simulink library "DABLib"  (R2016b)
settings: Solver=VariableStepAuto  StartTime=0.0  StopTime=10.0  RelTol=1e-3
undefined symbols (not defined in the file or in its folder): ln, sgn
libraries: DABLib x53, simulink_extras x2, simulink x1
(part 3 of 3)

== system DABLib/DABLibUtil/CoreAct/Ps//X transducer Pneumatic servo-motor/Twisted servomotor's rod fault f8 ==
  note: Fault  f8
      | Twisted servomotor's fault
      | simulated as linear function of X
  Db[m] : Inport
  X[%] : Inport  Port=2
  f8<0,1> : Inport  Port=3
  " " : Fcn  Expr=u(1)*(1+u(2)*u(3)*(1-u(4)))
  "Deadband 0..0.0381m " : Saturate  UpperLimit=0.0381  LowerLimit=0
  "Fault streght saturation 0..100% " : Saturate  UpperLimit=1.0  LowerLimit=0
  Higher bound 0..0.0381 : Saturate  UpperLimit=0.0381  LowerLimit=0
  Hysteresis change range in [%] : Constant  Value=0.5
  Mux4 : Mux
  Dbf[m] : Outport
  wires:
  " "/1 -> "Deadband 0..0.0381m "/1
  X[%]/1 -> Mux4/4
  Mux4/1 -> " "/1
  "Deadband 0..0.0381m "/1 -> Dbf[m]/1
  "Fault streght saturation 0..100% "/1 -> Mux4/3
  f8<0,1>/1 -> "Fault streght saturation 0..100% "/1
  Higher bound 0..0.0381/1 -> Mux4/1
  Db[m]/1 -> Higher bound 0..0.0381/1
  Hysteresis change range in [%]/1 -> Mux4/2

== system DABLib/DABLibUtil/CoreAct/Ps//X transducer Pneumatic servo-motor/Valve clogging fault f1 ==
  note: Fault  f1
      | Valve clogging fault
  Hb[m] : Inport
  f1<0,1> : Inport  Port=2
  " " : Fcn  Expr=u(1)*(1-u(2))
  "Fault streght saturation 0..100% " : Saturate  UpperLimit=1.0  LowerLimit=0
  Higher bound limit 0..0.0381m : Saturate  UpperLimit=0.0381  LowerLimit=0
  "Higher bound limit 0..0.0381m " : Saturate  UpperLimit=0.0381  LowerLimit=0
  Mux4 : Mux  Inputs=2
  Hbf[m] : Outport
  wires:
  "Fault streght saturation 0..100% "/1 -> Mux4/2
  Higher bound limit 0..0.0381m/1 -> Mux4/1
  Hb[m]/1 -> Higher bound limit 0..0.0381m/1
  " "/1 -> "Higher bound limit 0..0.0381m "/1
  Mux4/1 -> " "/1
  "Higher bound limit 0..0.0381m "/1 -> Hbf[m]/1
  f1<0,1>/1 -> "Fault streght saturation 0..100% "/1

== system DABLib/DABLibUtil/CoreAct/Ps//X transducer Pneumatic servo-motor/Valve errossion fault f3 ==
  note: Fault  f3
      | Valve plug or valve seat
      | errosion fault
  Hb[m] : Inport
  f3<0,1> : Inport  Port=2
  " " : Fcn  Expr=u(1)*(1+u(2)*u(3))
  Errossion relative span : Constant  Value=0.1
  "Fault streght saturation 0..100% " : Saturate  UpperLimit=1.0  LowerLimit=-1.0
  Higher bound limit 0..0.0381m : Saturate  UpperLimit=0.0381  LowerLimit=0
  "Higher bound limit 0..inf " : Saturate  UpperLimit=inf  LowerLimit=0
  Mux4 : Mux  Inputs=3
  Hbf[m] : Outport
  wires:
  Errossion relative span/1 -> Mux4/2
  "Fault streght saturation 0..100% "/1 -> Mux4/3
  Higher bound limit 0..0.0381m/1 -> Mux4/1
  Hb[m]/1 -> Higher bound limit 0..0.0381m/1
  " "/1 -> "Higher bound limit 0..inf "/1
  Mux4/1 -> " "/1
  "Higher bound limit 0..inf "/1 -> Hbf[m]/1
  f3<0,1>/1 -> "Fault streght saturation 0..100% "/1

== system DABLib/DABLibUtil/CoreAct/Ps//X transducer Pneumatic servo-motor/WUT Backlash ==
  dead band : Inport
  signal : Inport  Port=2
  Hysteresis : Subsystem
  Memory1 : Memory
  WUT direction decoder : Subsystem
  output : Outport
  wires:
  Hysteresis/1(hysta) -> Memory1/1, output/1
  Memory1/1 -> Hysteresis/4(history)
  dead band/1 -> Hysteresis/3(h_band)
  WUT direction decoder/1(direction) -> Hysteresis/2(x_dir)
  signal/1 -> Hysteresis/1(x), WUT direction decoder/1("signal ")

== system DABLib/DABLibUtil/CoreAct/Water flow control valve/Equipercentage rated flow coefficient ==
  note: Equipercentage rated flow
      | coefficient
  X[%] : Inport
  " 1" : Sum  Inputs=+-  SaturateOnIntegerOverflow=on  InputSameDT=on  OutDataTypeStr=Inherit: Same as first input
  " Valve Kv exponent" : Constant  Value=5
  Comparator : RelationalOperator  Operator=>  RndMeth=Nearest  InputSameDT=on
  End of equipercentage characteristics : Constant  Value=0.975
  Mux8 : Mux  Inputs=2
  Mux9 : Mux
  Rated flow coefficient Kv[%]=f(X[%]) Equipercentage part : Fcn  Expr=exp(u(2)*(1-u(1)))/exp(u(2))
  Rated flow coefficient Kv[%]=f[X[%]) Linear part : Fcn  Expr=u(2)*(u(4)-u(3))*(u(1)/(1-u(3)))
  Saturation 0..100% : Saturate  UpperLimit=1.00  LowerLimit=0
  Saturation 0..97.5% : Saturate  UpperLimit=0.975  LowerLimit=0
  Saturation 97.5%..100% : Saturate  UpperLimit=1.000  LowerLimit=0.975
  Kvr[%] : Outport
  wires:
  Saturation 0..100%/1 -> Saturation 97.5%..100%/1, Saturation 0..97.5%/1
  X[%]/1 -> Saturation 0..100%/1
  " 1"/1 -> Kvr[%]/1
  Rated flow coefficient Kv[%]=f[X[%]) Linear part/1 -> " 1"/2
  Saturation 97.5%..100%/1 -> Mux9/4, Comparator/1
  End of equipercentage characteristics/1 -> Mux9/3, Comparator/2
  Rated flow coefficient Kv[%]=f(X[%]) Equipercentage part/1 -> " 1"/1, Mux9/1
  Comparator/1 -> Mux9/2
  Mux9/1 -> Rated flow coefficient Kv[%]=f[X[%]) Linear part/1
  Saturation 0..97.5%/1 -> Mux8/1
  " Valve Kv exponent"/1 -> Mux8/2
  Mux8/1 -> Rated flow coefficient Kv[%]=f(X[%]) Equipercentage part/1

== system DABLib/DABLibUtil/CoreAct/Water flow control valve/Errosion fault  f3 gaining Kvr  ==
  note: Fault  f3
      | Errossion fault
  Kvr[%] : Inport
  f3<0,1> : Inport  Port=2
  " " : Fcn  Expr=u(1)*(1+u(2)*u(3))
  "Fault streght saturation 0..100% " : Saturate  UpperLimit=1.0  LowerLimit=0.0
  Mux4 : Mux  Inputs=3
  "Relative Kvr saturation 0..100% " : Saturate  UpperLimit=1.0  LowerLimit=0.0
  "Seat errosion relative span " : Constant  Value=0.10
  Kvrf[%] : Outport
  wires:
  "Relative Kvr saturation 0..100% "/1 -> Kvrf[%]/1
  " "/1 -> "Relative Kvr saturation 0..100% "/1
  "Seat errosion relative span "/1 -> Mux4/2
  "Fault streght saturation 0..100% "/1 -> Mux4/3
  f3<0,1>/1 -> "Fault streght saturation 0..100% "/1
  Kvr[%]/1 -> Mux4/1
  Mux4/1 -> " "/1

== system DABLib/DABLibUtil/CoreAct/Water flow control valve/Errossion fault  f3 X negative offset ==
  note: Fault  f3
      | Errossion fault
  X[%] : Inport
  f3<0,1> : Inport  Port=2
  " " : Fcn  Expr=u(1)-u(2)*u(3)
  "Fault range " : Constant  Value=0.10
  "Fault streght saturation 0..100% " : Saturate  UpperLimit=1.0  LowerLimit=0.0
  Mux4 : Mux  Inputs=3
  "Relative Xf saturation 0..100% " : Saturate  UpperLimit=1.0  LowerLimit=0.0
  Xf[%] : Outport
  wires:
  "Relative Xf saturation 0..100% "/1 -> Xf[%]/1
  " "/1 -> "Relative Xf saturation 0..100% "/1
  "Fault range "/1 -> Mux4/2
  "Fault streght saturation 0..100% "/1 -> Mux4/3
  f3<0,1>/1 -> "Fault streght saturation 0..100% "/1
  X[%]/1 -> Mux4/1
  Mux4/1 -> " "/1

== system DABLib/DABLibUtil/CoreAct/Water flow control valve/Internal leakage fault  f6 additive fault ==
  note: Fault  f6
      | Internal leakage fault
      | virtual Kv change
  Kvr[%] : Inport
  f6<0,1> : Inport  Port=2
  " " : Fcn  Expr=u(1)+u(2)*u(3)
  Fault range in [%] <0..1> : Constant  Value=0.10
  "Fault streght saturation 0..100% " : Saturate  UpperLimit=1.0  LowerLimit=0.0
  Mux4 : Mux  Inputs=3
  Kvrf[%] : Outport
  wires:
  Fault range in [%] <0..1>/1 -> Mux4/2
  "Fault streght saturation 0..100% "/1 -> Mux4/3
  " "/1 -> Kvrf[%]/1
  f6<0,1>/1 -> "Fault streght saturation 0..100% "/1
  Kvr[%]/1 -> Mux4/1
  Mux4/1 -> " "/1

== system DABLib/DABLibUtil/CoreAct/Water flow control valve/Sedimentation fault  f2 Kvr lowering ==
  note: Fault  f2
      | Sedimentation fault
  Kvr[%] : Inport
  f2<0,1> : Inport  Port=2
  " " : Fcn  Expr=u(1)*(1-u(2)*u(3))
  "Fault streght saturation 0..100% " : Saturate  UpperLimit=1.0  LowerLimit=0.0
  Mux4 : Mux  Inputs=3
  "Relative Kvr saturation 0..100% " : Saturate  UpperLimit=1.0  LowerLimit=0.0
  "Seat sedimentation relative span " : Constant  Value=0.20
  Kvrf[%] : Outport
  wires:
  "Relative Kvr saturation 0..100% "/1 -> Kvrf[%]/1
  " "/1 -> "Relative Kvr saturation 0..100% "/1
  "Seat sedimentation relative span "/1 -> Mux4/2
  "Fault streght saturation 0..100% "/1 -> Mux4/3
  f2<0,1>/1 -> "Fault streght saturation 0..100% "/1
  Kvr[%]/1 -> Mux4/1
  Mux4/1 -> " "/1

== system DABLib/DABLibUtil/CoreAct/Water flow control valve/Sedimentation fault  f2 X positive offset ==
  note: Fault  f2
      | Sedimentation fault
  X[%] : Inport
  f2<0,1> : Inport  Port=2
  " " : Fcn  Expr=u(1)+u(2)*u(3)
  "Fault range " : Constant  Value=0.20
  "Fault streght saturation 0..100% " : Saturate  UpperLimit=1.0  LowerLimit=0.0
  Mux4 : Mux  Inputs=3
  "Relative Xf saturation 0..100% " : Saturate  UpperLimit=1.0  LowerLimit=0.0
  Xf[%] : Outport
  wires:
  "Relative Xf saturation 0..100% "/1 -> Xf[%]/1
  " "/1 -> "Relative Xf saturation 0..100% "/1
  "Fault range "/1 -> Mux4/2
  "Fault streght saturation 0..100% "/1 -> Mux4/3
  f2<0,1>/1 -> "Fault streght saturation 0..100% "/1
  X[%]/1 -> Mux4/1
  Mux4/1 -> " "/1

== system DABLib/DABLibUtil/CoreAct/Water flow control valve/water specific gravity ==
  note: Water specific gravity versus temperature and pressure
  P[Pa] : Inport
  T[C] : Inport  Port=2
  1-C*P : Fcn  Expr=1-u
  C*P : Product  SaturateOnIntegerOverflow=on  RndMeth=Zero  InputSameDT=on  OutDataTypeStr=Inherit: Same as first input
  Switch : Switch  Threshold=30  SaturateOnIntegerOverflow=on  InputSameDT=on
  Temperature range 0..110C : Saturate  UpperLimit=110  LowerLimit=0
  Water compessibility coefficient : Lookup  InputValues=[0 10 20 50 110]  Table="[5.26e-10 5.02e-10  4.81e-10 4.69e-10 4.42e-10]"  SaturateOnIntegerOverflow=on
  "ro(T)/(1-C(T)*P) " : Product  Inputs=*/  SaturateOnIntegerOverflow=on  RndMeth=Zero  InputSameDT=on  OutDataTypeStr=Inherit: Same as first input
  ro[kg/m^3] t<0..40>C : Fcn  Expr=1000-(((u-4)^2)/503570)*(u+283)*1000/(u+67.2)
  ro[kg/m^3] t<25..100>C : Fcn  Expr=1000-((((u-4)^2)/466700)*(u+273)*1000*(350-u))/((u+67)*(365-u))
  ro[kg/m^3] : Outport
  wires:
  "ro(T)/(1-C(T)*P) "/1 -> ro[kg/m^3]/1
  1-C*P/1 -> "ro(T)/(1-C(T)*P) "/2
  Switch/1 -> "ro(T)/(1-C(T)*P) "/1
  C*P/1 -> 1-C*P/1
  Water compessibility coefficient/1 -> C*P/1
  ro[kg/m^3] t<25..100>C/1 -> Switch/1
  ro[kg/m^3] t<0..40>C/1 -> Switch/3
  Temperature range 0..110C/1 -> Water compessibility coefficient/1, Switch/2, ro[kg/m^3] t<0..40>C/1, ro[kg/m^3] t<25..100>C/1
  T[C]/1 -> Temperature range 0..110C/1
  P[Pa]/1 -> C*P/2

== system DABLib/PICalc/Zones Selection/Stop-watch 1st/Stop-watch ==
  Trigger : TriggerPort  VariantControl=Variant  ShowOutputPort=on
  Digital Clock : DigitalClock  SampleTime=-1
  t(k) : Outport  InitialOutput=-1
  TR : Outport  Port=2  InitialOutput=0
  wires:
  Digital Clock/1 -> t(k)/1
  Trigger/1 -> TR/1

== system DABLib/DABLibUtil/CoreAct/Positioner feedback/WUT Backlash/Hysteresis ==
  x : Inport
  x_dir : Inport  Port=2
  h_band : Inport  Port=3
  history : Inport  Port=4
  Gain : Gain  Gain=0.5  SaturateOnIntegerOverflow=on  OutDataTypeStr=Inherit: Same as input  ParamDataTypeStr=Inherit: Same as input
  MinMax : MinMax  Inputs=2  SaturateOnIntegerOverflow=on  InputSameDT=on
  MinMax1 : MinMax  Function=max  Inputs=2  SaturateOnIntegerOverflow=on  InputSameDT=on
  Switch : Switch  Threshold=0.5  SaturateOnIntegerOverflow=on  InputSameDT=on
  sum : Sum  Inputs=+-  SaturateOnIntegerOverflow=on  InputSameDT=on  OutDataTypeStr=Inherit: Same as first input
  sum1 : Sum  SaturateOnIntegerOverflow=on  InputSameDT=on  OutDataTypeStr=Inherit: Same as first input
  hysta : Outport  InitialOutput=0
  wires:
  Gain/1 -> sum/2, sum1/2
  sum1/1 -> MinMax/1  "y"
  history/1 -> MinMax/2, MinMax1/2
  h_band/1 -> Gain/1
  Switch/1 -> hysta/1
  sum/1 -> MinMax1/1  "z"
  x_dir/1 -> Switch/2
  MinMax1/1 -> Switch/1
  MinMax/1 -> Switch/3
  x/1 -> sum/1, sum1/1

== system DABLib/DABLibUtil/CoreAct/Positioner feedback/WUT Backlash/WUT direction decoder ==
  note: du/dt
  "signal " : Inport
  Memory : Memory
  Sum2 : Sum  Inputs=+-  SaturateOnIntegerOverflow=on  InputSameDT=on  OutDataTypeStr=Inherit: Same as first input
  Terminator : Terminator
  Zero cross : HitCross  HitCrossingDirection=falling
  "Zero cross " : HitCross  HitCrossingDirection=rising
  direction FF : simulink_extras/Flip Flops/S-R Flip-Flop  initial_condition=0
  direction : Outport
  wires:
  direction FF/2 -> Terminator/1
  "signal "/1 -> Memory/1, Sum2/1
  direction FF/1 -> direction/1  "u2"
  Sum2/1 -> "Zero cross "/1, Zero cross/1
  Memory/1 -> Sum2/2
  Zero cross/1 -> direction FF/2
  "Zero cross "/1 -> direction FF/1

== system DABLib/DABLibUtil/CoreAct/Ps//X transducer Pneumatic servo-motor/WUT Backlash/Hysteresis ==
  x : Inport
  x_dir : Inport  Port=2
  h_band : Inport  Port=3
  history : Inport  Port=4
  Gain : Gain  Gain=0.5  SaturateOnIntegerOverflow=on  OutDataTypeStr=Inherit: Same as input  ParamDataTypeStr=Inherit: Same as input
  MinMax : MinMax  Inputs=2  SaturateOnIntegerOverflow=on  InputSameDT=on
  MinMax1 : MinMax  Function=max  Inputs=2  SaturateOnIntegerOverflow=on  InputSameDT=on
  Switch : Switch  Threshold=0.5  SaturateOnIntegerOverflow=on  InputSameDT=on
  sum : Sum  Inputs=+-  SaturateOnIntegerOverflow=on  InputSameDT=on  OutDataTypeStr=Inherit: Same as first input
  sum1 : Sum  SaturateOnIntegerOverflow=on  InputSameDT=on  OutDataTypeStr=Inherit: Same as first input
  hysta : Outport  InitialOutput=0
  wires:
  Gain/1 -> sum/2, sum1/2
  sum1/1 -> MinMax/1  "y"
  history/1 -> MinMax/2, MinMax1/2
  h_band/1 -> Gain/1
  Switch/1 -> hysta/1
  sum/1 -> MinMax1/1  "z"
  x_dir/1 -> Switch/2
  MinMax1/1 -> Switch/1
  MinMax/1 -> Switch/3
  x/1 -> sum/1, sum1/1

== system DABLib/DABLibUtil/CoreAct/Ps//X transducer Pneumatic servo-motor/WUT Backlash/WUT direction decoder ==
  note: du/dt
  "signal " : Inport
  Memory : Memory
  Sum2 : Sum  Inputs=+-  SaturateOnIntegerOverflow=on  InputSameDT=on  OutDataTypeStr=Inherit: Same as first input
  Terminator : Terminator
  Zero cross : HitCross  HitCrossingDirection=falling
  "Zero cross " : HitCross  HitCrossingDirection=rising
  direction FF : simulink_extras/Flip Flops/S-R Flip-Flop  initial_condition=0
  direction : Outport
  wires:
  direction FF/2 -> Terminator/1
  "signal "/1 -> Memory/1, Sum2/1
  direction FF/1 -> direction/1  "u2"
  Sum2/1 -> "Zero cross "/1, Zero cross/1
  Memory/1 -> Sum2/2
  Zero cross/1 -> direction FF/2
  "Zero cross "/1 -> direction FF/1
